simulink model "AirRefueling_Platform_IBVS"  (R2022b)
settings: Solver=FixedStepAuto  StartTime=0.0  StopTime=70  FixedStep=0.02  RelTol=1e-5  AbsTol=1e-4  EnableMultiTasking=on
InitFcn:
  | F16_Init
values from neighbouring files (symbols this model uses):
  airSpeed = 393.720000000000    (= 393.72)    [F16_Init.m]    (also in Initialization.m)
  alpha0 = trimAlpha*180/pi    (= 6.62393794015)    [F16_Init.m]    (also in Initialization.m)
  altitude = 9843    [F16_Init.m]    (also in Initialization.m)
  b_ref = 30.0    (= 30)    [F16_Init.m]    (also in Initialization.m)
  C2m = [C(1,:) ... (first row only)    [F16_Init.m]    (also in Initialization.m)
  d_f_rc = [3.75;0;-0.86]    [F16_Init.m]
  d_pr_rc = [6.06;0.54;-0.86]    [F16_Init.m]
  dLEF = 0    [F16_Init.m]    (also in Initialization.m)
  fi_flag = 1    [F16_Init.m]    (also in Initialization.m)
  Kc = [ ... (first row only)    [F16_Init.m]    (also in Initialization.m)
  Ki = zeros(4,3)    [F16_Init.m]    (also in Initialization.m)
  Kp = zeros(4,18)    [F16_Init.m]    (also in Initialization.m)
  mass = 636.94    [F16_Init.m]    (also in Initialization.m)
  p0_rc = [-14.35-6.06-6;-0.54-(2);5.12+0.86-(-2)]    [F16_Init.m]
  q = zeros(N,1)    [hose3D_n_air_Fv_correction.m]
  trim_ail = 0.00874607850103852    (= 0.00874607850104)    [F16_Init.m]    (also in Initialization.m)
  trim_control = [trim_thrust;trim_ele;trim_ail;trim_rud]    [F16_Init.m]    (also in Initialization.m)
  trim_ele = -2.97973164860638    (= -2.97973164861)    [F16_Init.m]    (also in Initialization.m)
  trim_rud = 0.0680302158182712    (= 0.0680302158183)    [F16_Init.m]    (also in Initialization.m)
  trim_state1 = [trim_state;0;0;0;0;0;0]    [F16_Init.m]    (also in Initialization.m)
  trim_thrust = 2279.08519954656    (= 2279.08519955)    [F16_Init.m]    (also in Initialization.m)
undefined symbols (not defined in the file or in its folder): F, gray, MIL, vt0
libraries: aerolibconvert2 x4, aerolibasang x4, aerolibwind2 x3, visionmorphops x3, vrlib x2, aerolibobsolete x2, simulink x1, visionconversions x1, visiongeotforms x1, aerolibatmos2 x1, aerolibadyn x1, aerolibanimutils x1
(part 1 of 2)
settings Model: Creator=WhisPer  LastModifiedBy=Jinrui
settings SolverCC: AutoScaleAbsTol=off  AlgebraicLoopSolver=TrustRegion
settings DataIOCC: LimitDataPoints=on  SaveFormat=Array  ReturnWorkspaceOutputs=off
settings OptimizationCC: LifeSpan=inf
settings DebuggingCC: UnderspecifiedInitializationDetection=Classic  MergeDetectMultiDrivingBlocksExec=none  SolverPrmCheckMsg=warning  UnconnectedInputMsg=warning  UnconnectedOutputMsg=warning  UnconnectedLineMsg=warning  StateNameClashWarn=warning  SFUnexpectedBacktrackingDiag=warning  SFNoUnconditionalDefaultTransitionDiag=warning  SFExecutionAtInitializationDiag=none  SFMachineParentedDataDiag=warning  ArithmeticOperatorsInVariantConditions=warning
settings HardwareCC: ProdBitPerPointer=32  ProdBitPerSizeT=32  ProdBitPerPtrDiffT=32  ProdLargestAtomicFloat=None  ProdIntDivRoundTo=Undefined  ProdEndianess=Unspecified  ProdWordSize=32  ProdHWDeviceType=32-bit Generic
settings ModelReferenceCC: EnableRefExpFcnMdlSchedulingChecks=on  PropagateSignalLabelsOutOfModel=off
settings SFSimCC: SimUseLocalCustomCode=off  CustomCodeUndefinedFunction=UseInterfaceOnly
settings RTWCC: RTWUseLocalCustomCode=off  DLArmComputeVersion=19.05
settings CodeAppCC: StateflowObjectComments=on
settings GRTTargetCC: TargetLangStandard=C89/C90 (ANSI)
settings ConfigComp: CovMetricSettings=dw  CovSaveCumulativeToWorkspaceVar=on  CovSaveSingleToWorkspaceVar=on  CovExternalEMLEnable=off

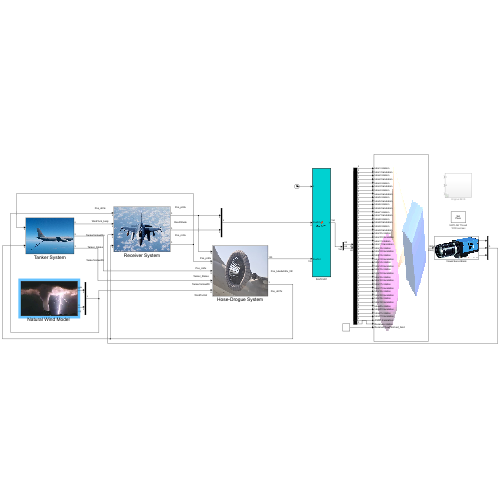
[thumbnail: Simulink's stored preview of the top-level diagram]
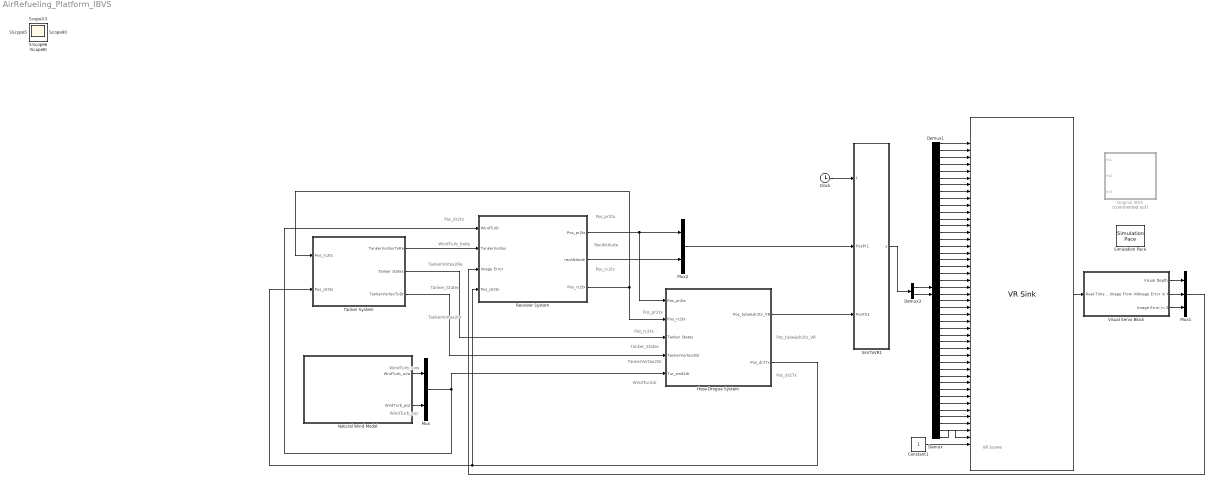
== system AirRefueling_Platform_IBVS ==
  note: Pos_pr2tx
  note: VR Scene
  note: RecAttitude
  note: WindTurb_uvw
  note: WindTurb_pqr
  note: Pos_dr2Tx
  note: Pos_tube&dr2tx_VR
  note: WindTur2dr
  note: Pos_pr2tx
  note: WindTurb_body
  note: Pos_dr2tx
  note: Pos_rc2tx
  note: TankerVortex2Re
  note: TankerVortex2Dr
  note: Tanker_States
  note: Tanker_States
  note: TankerVortex2Dr
  note: Pos_rc2tx
  " " : vrlib/VR Sink  InstantiateOnLoad=on  SampleTime=-1  ViewEnable=on  RemoteChange=off  RemoteView=off  FieldsWritten=tube1.rotation.4.1.1.double#tube1.translation.3.1.1.double#tube2.rotation.4.1.1.double#tube2.translation.3.1.1.double#tube3.rotation.4.1.1.double#tube3.translation.3.1.1.double#tube4.rotation.4.1.1.double#tube4.translation.3.1.1.double#tube5.rotation.4.1.1.double#tube5.translation.3.1.1.double#tube6.rotation.4.1.1.double#tube6.translation.3.1.1.double#tube7.rotation.4.1.1.double#tube7.translation.3.1.1.double#tube8.rotation.4.1.1.double#tube8.translation.3.1.1.double#tube9.rotation.4.1.1.double#tube9.translation.3.1.1.double#tube10.rotation.4.1.1.double#tube10.translation.3.1.1.double#tube11.rotation.4.1.1.double#tube11.translation.3.1.1.double#tube12.rotation.4.1.1.double#tube12.translation.3.1.1.double#tube13.rotation.4.1.1.double#tube13.translation.3.1.1.double#tube14.rotation.4.1.1.double#tube14.translation.3.1.1.double#tube15.rotation.4.1.1.double#tube15.translation.3.1.1.double#tube16.rotation.4.1.1.double#tube16.translation.3.1.1.double#tube17.rotation.4.1.1.double#tube17.translation.3.1.1.double#tube18.rotation.4.1.1.double#tube18.translation.3.1.1.double#tube19.rotation.4.1.1.double#tube19.translation.3.1.1.double#tube20.rotation.4.1.1.double#tube20.translation.3.1.1.double#tube21.rotation.4.1.1.double#tube21.translation.3.1.1.double#ASDD.translation.3.1.1.double#Receiver.rotation.4.1.1.double#ReceiverViewPoint.set_bind.1.1.1.logical  WorldFileName=AirRefuelingTubeSim_Image.WRL  AutoView=off  VideoDimensions=[200 320]  AllowVariableSize=off  FigureProperties="{'Position', 'Name', 'Viewpoint', 'CameraBound', 'CameraDirection', 'CameraPosition', 'CameraUpVector', 'ZoomFactor', 'Antialiasing', 'Headlight', 'Lighting', 'NavPanel', 'Sound', 'StatusBar', 'Stereo3D', 'Stereo3DCameraOffset', 'Stereo3DHIT', 'ToolBar', 'Textures', 'Transparency', 'Triad', 'Wireframe', 'NavZones', 'NavMode', 'NavSpeed', 'CaptureFileFormat', 'CaptureFileName', 'Record2DCompressMethod', 'Record2DCompressQuality', 'Record2D', 'Record2DFileName', 'Record2DFPS'; [3.0000000000000000e+01   6.0000000000000000e+01   3.2000000000000000e+02   2.0000000000000000e+02], '', 'Receive1', 'on', [-9.4108294567116141e-02   0.0000000000000000e+00  -9.9556196637560879e-01], [-2.1616954617207307e-01   0.0000000000000000e+00  -1.0387194196845528e+00], [0.0000000000000000e+00   1.0000000000000000e+00   0.0000000000000000e+00], [1.0000000000000000e+00], 'on', 'on', 'on', 'none', 'on', 'off', 'off', [1.0000000149011612e-01], [0.0000000000000000e+00], 'off', 'on', 'on', 'none', 'off', 'off', 'walk', 'normal', 'tif', '%f_anim_%n.tif', 'auto', [7.5000000000000000e+01], 'off', '***video***', 'auto'}"
  Clock : Clock
  Constant1 : Constant
  Demux : Demux  Outputs=22
  Demux1 : Demux  Outputs=22
  Demux3 : Demux  Outputs=[88,66]
  Hose-Drogue System : Subsystem
      mask Display: image(imread('Icon\drogue.jpg'))
  Mux : Mux  Inputs=2
  Mux1 : Mux  Inputs=3
  Mux2 : Mux  Inputs=2
  "Natural Wind Model " : Subsystem
      mask Display: image(imread('Icon\Enviroment.jpg'))
  Original IBVS : Subsystem  Commented=on
  Receiver System : Subsystem
      mask Display: image(imread('Icon\f16thumb.jpg'))
  SimToVR1 : MATLAB Function  TreatAsAtomicUnit=on
  Simulation Pace : aerolibanimutils/Simulation Pace  SimulationPace=1000  SleepMode=MATLAB Thread  OutputPaceError=off  SampleTime=-1
  Tanker System : Subsystem
      mask Display: image(imread('Icon\tanker.jpg'))
  Visual Servo Block : Subsystem
      mask Display: image('icon/camera.jpg');
  Scope{,1,3..34} (34 alike) : Scope
  wires:
  Receiver System/1(Pos_pr2tx) -> Mux2/1, Hose-Drogue System/1(Pos_pr2tx)
  Hose-Drogue System/2(Pos_dr2Tx) -> Tanker System/2(Pos_dr2tx), Receiver System/4(Pos_dr2tx)
  Mux/1 -> Receiver System/1(WindTurb), Hose-Drogue System/5(Tur_wnd2dr)
  Receiver System/2(recAttitude) -> Mux2/2
  Hose-Drogue System/1(Pos_tube&dr2tx_VR) -> SimToVR1/3(PosTb1)
  Mux2/1 -> SimToVR1/2(PosPr1)
  "Natural Wind Model "/1(WndTurb_uvw) -> Mux/1
  "Natural Wind Model "/2(WndTurb_pqr) -> Mux/2
  Demux3/2 -> Demux/1
  Demux/22 -> " "/43
  Demux1/22 -> " "/44
  Demux3/1 -> Demux1/1
  Tanker System/2(Tanker states) -> Hose-Drogue System/3(Tanker States)
  Tanker System/3(TankerVortexToDr) -> Hose-Drogue System/4(TankerVortex2Dr)
  Tanker System/1(TankerVortexToRe) -> Receiver System/2(TankerVortex)
  Receiver System/3(Pos_rc2tx) -> Tanker System/1(Pos_rc2tx), Hose-Drogue System/2(Pos_rc2tx)
  Clock/1 -> SimToVR1/1(t)
  Demux1/1 -> " "/1
  Demux/1 -> " "/2
  Demux1/2 -> " "/3
  Demux/2 -> " "/4
  Demux1/3 -> " "/5
  Demux/3 -> " "/6
  Demux1/4 -> " "/7
  Demux/4 -> " "/8
  Demux1/5 -> " "/9
  Demux/5 -> " "/10
  Demux1/6 -> " "/11
  Demux/6 -> " "/12
  Demux1/7 -> " "/13
  Demux/7 -> " "/14
  Demux1/8 -> " "/15
  Demux/8 -> " "/16
  Demux1/9 -> " "/17
  Demux/9 -> " "/18
  Demux1/10 -> " "/19
  Demux/10 -> " "/20
  Demux1/11 -> " "/21
  Demux/11 -> " "/22
  Demux1/12 -> " "/23
  Demux/12 -> " "/24
  Demux1/13 -> " "/25
  Demux/13 -> " "/26
  Demux1/14 -> " "/27
  Demux/14 -> " "/28
  Demux1/15 -> " "/29
  Demux/15 -> " "/30
  Demux1/16 -> " "/31
  Demux/16 -> " "/32
  Demux1/17 -> " "/33
  Demux/17 -> " "/34
  Demux1/18 -> " "/35
  Demux/18 -> " "/36
  Demux1/19 -> " "/37
  Demux/19 -> " "/38
  Demux1/20 -> " "/39
  Demux/20 -> " "/40
  Demux1/21 -> " "/41
  Demux/21 -> " "/42
  Constant1/1 -> " "/45
  " "/1 -> Visual Servo Block/1(Real-Time Image From VR)
  Visual Servo Block/1(Visual Depth) -> Mux1/1
  Visual Servo Block/2(Image Error in Y) -> Mux1/2
  Visual Servo Block/3(Image Error in Z) -> Mux1/3
  Mux1/1 -> Receiver System/3(Image Error)
  SimToVR1/1(y) -> Demux3/1

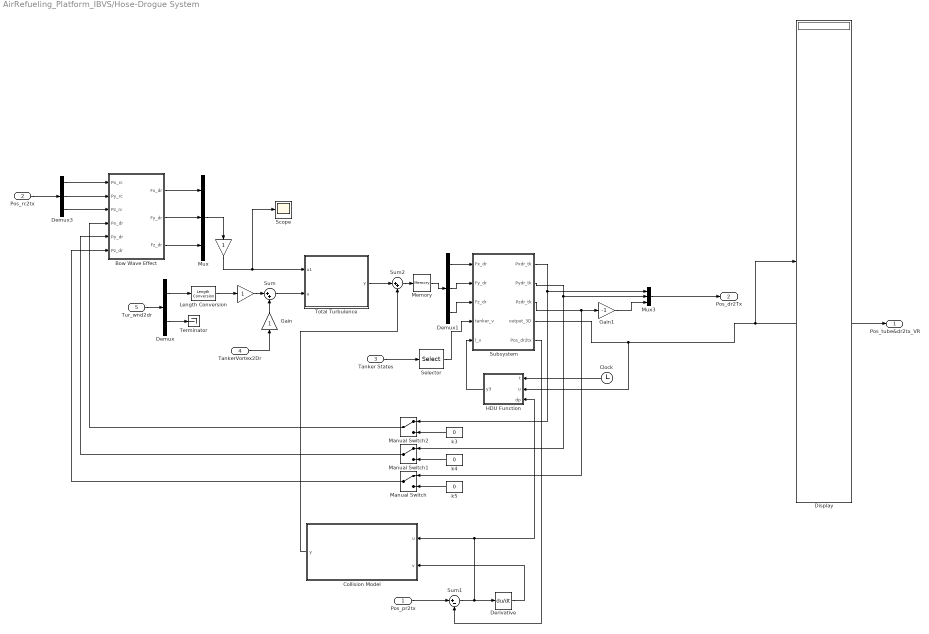
== system AirRefueling_Platform_IBVS/Hose-Drogue System ==
  Pos_pr2tx : Inport
  Pos_rc2tx : Inport  Port=2
  Tanker States : Inport  Port=3
  TankerVortex2Dr : Inport  Port=4
  Tur_wnd2dr : Inport  Port=5
  " " : Gain
  "  " : Gain
  Bow Wave Effect : Subsystem
  Clock : Clock
  Collision Model : MATLAB Function  TreatAsAtomicUnit=on
  Demux : Demux  Outputs=2
  Demux1 : Demux  Outputs=3
  Demux3 : Demux  Outputs=3
  Derivative : Derivative
  Display : Display
  Gain : Gain
  Gain1 : Gain  Gain=-1
  HDU Function : MATLAB Function  TreatAsAtomicUnit=on
  Length Conversion : aerolibconvert2/Length Conversion  IU=ft  OU=m
  Manual Switch : ManualSwitch
  Manual Switch1 : ManualSwitch
  Manual Switch2 : ManualSwitch
  Memory : Memory
  Mux : Mux  Inputs=3
  Mux3 : Mux  Inputs=3
  Scope : Scope
  Selector : Selector  InputPortWidth=9  IndexOptions=Index vector (dialog)  Indices=[4 5 6]  OutputSizes=1
  Subsystem : Subsystem
  Sum : Sum  Inputs=|++
  Sum1 : Sum  Inputs=|+-
  Sum2 : Sum  Inputs=|++
  Terminator : Terminator
  "Total Turbulence  " : MATLAB Function  TreatAsAtomicUnit=on
  k3 : Constant  Value=0
  k4 : Constant  Value=0
  k5 : Constant  Value=0
  Pos_tube&dr2tx_VR : Outport
  Pos_dr2Tx : Outport  Port=2
  wires:
  Mux/1 -> "  "/1
  TankerVortex2Dr/1 -> Gain/1
  Demux/1 -> Length Conversion/1
  Demux1/3 -> Subsystem/3(Fz_dr)
  Demux1/2 -> Subsystem/2(Fy_dr)
  Demux1/1 -> Subsystem/1(Fx_dr)
  Demux/2 -> Terminator/1
  Tur_wnd2dr/1 -> Demux/1
  Pos_rc2tx/1 -> Demux3/1
  Bow Wave Effect/3(Fz_dr) -> Mux/3
  Sum/1 -> "Total Turbulence  "/2(u)
  Bow Wave Effect/2(Fy_dr) -> Mux/2
  Bow Wave Effect/1(Fx_dr) -> Mux/1
  Demux3/1 -> Bow Wave Effect/1(Px_rc)
  k4/1 -> Manual Switch1/2
  Manual Switch1/1 -> Bow Wave Effect/5(Py_dr)
  Manual Switch2/1 -> Bow Wave Effect/4(Px_dr)
  k5/1 -> Manual Switch/2
  k3/1 -> Manual Switch2/2
  Mux3/1 -> Pos_dr2Tx/1
  Manual Switch/1 -> Bow Wave Effect/6(Pz_dr)
  Subsystem/2(Pydr_tk) -> Manual Switch1/1, Mux3/2
  Subsystem/1(Pxdr_tk) -> Manual Switch2/1, Mux3/1
  Gain1/1 -> Mux3/3
  Subsystem/3(Pzdr_tk) -> Gain1/1, Manual Switch/1
  Demux3/3 -> Bow Wave Effect/3(Pz_rc)
  Demux3/2 -> Bow Wave Effect/2(Py_rc)
  "Total Turbulence  "/1(y) -> Sum2/1
  Subsystem/4(output_3D) -> Display/1, Pos_tube&dr2tx_VR/1, HDU Function/2(u)
  Gain/1 -> Sum/2
  " "/1 -> Sum/1
  "  "/1 -> Scope/1, "Total Turbulence  "/1(u1)
  Length Conversion/1 -> " "/1
  Tanker States/1 -> Selector/1
  Sum1/1 -> HDU Function/3(dp), Collision Model/1(u), Derivative/1
  Derivative/1 -> Collision Model/2(v)
  Sum2/1 -> Memory/1
  Collision Model/1(y) -> Sum2/2
  Selector/1 -> Subsystem/4(tanker_v)
  Subsystem/5(Pos_dr2tx) -> Sum1/2
  Memory/1 -> Demux1/1
  Clock/1 -> HDU Function/1(t)
  HDU Function/1(y3) -> Subsystem/5(l_v)
  Pos_pr2tx/1 -> Sum1/1

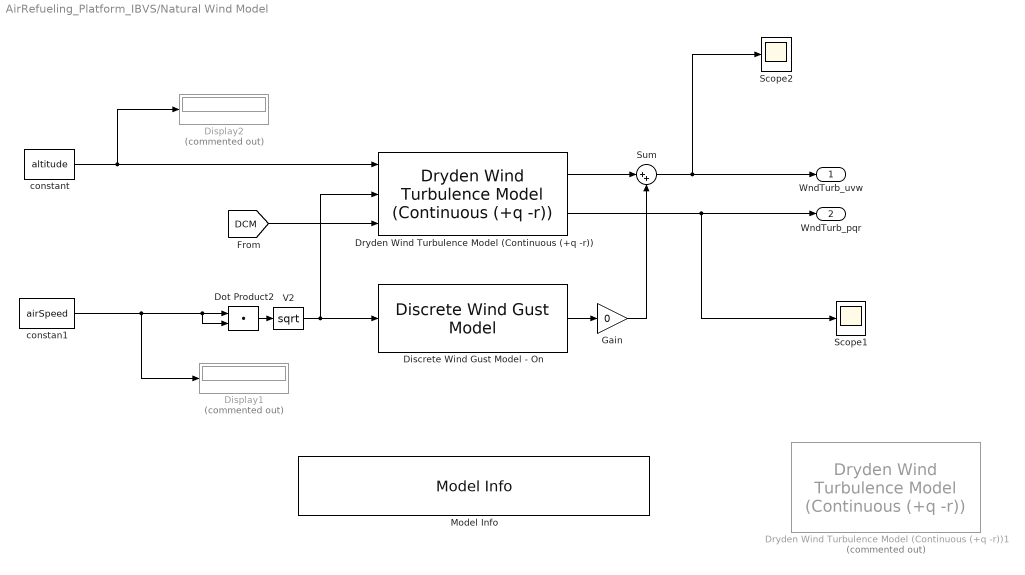
== system AirRefueling_Platform_IBVS/Natural Wind Model  ==
  Discrete Wind Gust Model - On : aerolibwind2/Discrete Wind Gust Model  units=English (Velocity in ft/s)  Gx=on  Gy=on  Gz=on  t_0=20  d_m=[120 120 80]  v_m=[0 0 0]
  Display1 : Display  Commented=on
  Display2 : Display  Commented=on
  Dot Product2 : DotProduct  SaturateOnIntegerOverflow=on  InputSameDT=off  OutDataTypeStr=Inherit: Inherit via internal rule
  Dryden Wind Turbulence Model (Continuous (+q -r)) : aerolibwind2/Dryden Wind Turbulence Model  (Continuous (+q -r))  units=English (Velocity in ft/s)  spec=MIL-F-8785C  model=Continuous Dryden (+q -r)  W20=5  Wdeg=0  TurbProb=2x10^-1  L_high=533.4  Wingspan=4  ts=0.02  Seed=[23341 23342 23343 23344]  T_on=on
  Dryden Wind Turbulence Model (Continuous (+q -r))1 : aerolibwind2/Dryden Wind Turbulence Model  (Continuous (+q -r))  Commented=on  units=English (Velocity in ft/s)  spec=MIL-F-8785C  model=Continuous Dryden (+q -r)  W20=5  Wdeg=0  TurbProb=2x10^-1  L_high=533.5  Wingspan=6  ts=0.02  Seed=1+fix(3650*rand(1,4))  T_on=on
  Gain : Gain  Gain=0
  Model Info : simulink/Model-Wide Utilities/Model Info  Frame=on  DisplayStringWithTags=|  HorizontalTextAlignment=Center  LeftAlignmentValue=0.5
      | The resultant mean wind speed and angular rates is in the body-fixed axis. 
      | The simulation parameter is set to
      | altitude:3000m
      | airspeed:120m/s
  Scope1 : Scope
  Scope2 : Scope
  Sum : Sum  Inputs=|++  InputSameDT=on  SaturateOnIntegerOverflow=on  OutDataTypeStr=Inherit: Same as first input
  V2 : Math  Operator=sqrt  SignedPower=on
  constan1 : Constant  Value=airSpeed
  constant : Constant  Value=altitude
  WndTurb_uvw : Outport
  WndTurb_pqr : Outport  Port=2
  wires:
  V2/1 -> Dryden Wind Turbulence Model (Continuous (+q -r))/2, Discrete Wind Gust Model - On/1
  Dot Product2/1 -> V2/1
  constan1/1 -> Dot Product2/1, Dot Product2/2, Display1/1
  Discrete Wind Gust Model - On/1 -> Gain/1
  Dryden Wind Turbulence Model (Continuous (+q -r))/1 -> Sum/1
  constant/1 -> Dryden Wind Turbulence Model (Continuous (+q -r))/1, Display2/1
  [DCM] -> Dryden Wind Turbulence Model (Continuous (+q -r))/3
  Sum/1 -> WndTurb_uvw/1, Scope2/1
  Dryden Wind Turbulence Model (Continuous (+q -r))/2 -> Scope1/1, WndTurb_pqr/1
  Gain/1 -> Sum/2

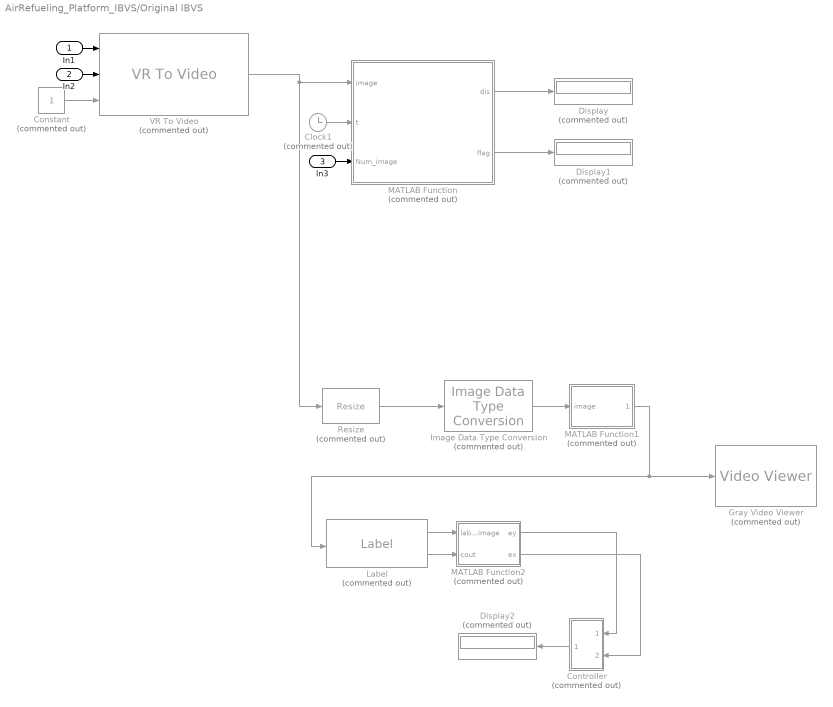
== system AirRefueling_Platform_IBVS/Original IBVS ==
  In1 : Inport
  In2 : Inport  Port=2
  In3 : Inport  Port=3
  Clock1 : Clock  Commented=on
  Constant : Constant  Commented=on
  Controller : Subsystem  Commented=on
  Display : Display  Commented=on
  Display1 : Display  Commented=on
  Display2 : Display  Commented=on
  Gray Video Viewer : VideoViewer  Commented=on  FigPos=[594 894 615 423]
  Image Data Type Conversion : visionconversions/Image Data Type Conversion  Commented=on  outDT=double  isSigned=on  wordLen=16  numFracBits=0
  Label : visionmorphops/Label  Commented=on  conn=8  output=Label matrix and number of labels  outType=Automatic  lastLabel=maximum value of the output data type
  MATLAB Function : MATLAB Function  Commented=on  TreatAsAtomicUnit=on
  MATLAB Function1 : MATLAB Function  Commented=on  TreatAsAtomicUnit=on
  MATLAB Function2 : MATLAB Function  Commented=on  TreatAsAtomicUnit=on
  Resize : visiongeotforms/Resize  Commented=on  specify=Output size as a percentage of input size  rfactor=[200 150]  outCols=25  outRows=25  outRowsCols=[25 35]  interp_method=Bilinear  antialias=on  useROI=off  roiFlag=off  prodOutputMode=Binary point scaling  prodOutputWordLength=32  prodOutputFracLength=10  roundingMode=Nearest  overflowMode=on
  VR To Video : vrlib/VR To Video  Commented=on  InstantiateOnLoad=on  SampleTime=0.01  ViewEnable=on  RemoteChange=off  RemoteView=off  FieldsWritten=Anigroup-1-Intrp7-transform.rotation.4.1.1.double#Anigroup-1-Intrp7-transform.translation.3.1.1.double#ReceiverViewPoint.set_bind.1.1.1.logical  WorldFileName=AirRefuelingTubeSim.WRL  AutoView=off  VideoDimensions=[200 320]  AllowVariableSize=off  FigureProperties="{'Position', 'Name', 'Viewpoint', 'CameraBound', 'CameraDirection', 'CameraPosition', 'CameraUpVector', 'ZoomFactor', 'Antialiasing', 'Headlight', 'Lighting', 'NavPanel', 'Sound', 'StatusBar', 'Stereo3D', 'Stereo3DCameraOffset', 'Stereo3DHIT', 'ToolBar', 'Textures', 'Transparency', 'Triad', 'Wireframe', 'NavZones', 'NavMode', 'NavSpeed', 'CaptureFileFormat', 'CaptureFileName', 'Record2DCompressMethod', 'Record2DCompressQuality', 'Record2D', 'Record2DFileName', 'Record2DFPS'; [3.0000000000000000e+01   6.0000000000000000e+01   3.2000000000000000e+02   2.0000000000000000e+02], '', 'Receive1', 'on', [0.0000000000000000e+00   0.0000000000000000e+00  -1.0000000000000000e+00], [0.0000000000000000e+00   0.0000000000000000e+00   0.0000000000000000e+00], [0.0000000000000000e+00   1.0000000000000000e+00   0.0000000000000000e+00], [1.0000000000000000e+00], 'on', 'on', 'on', 'none', 'on', 'off', 'off', [1.0000000149011612e-01], [0.0000000000000000e+00], 'off', 'on', 'on', 'none', 'off', 'off', 'walk', 'normal', 'tif', '%f_anim_%n.tif', 'auto', [7.5000000000000000e+01], 'off', '***video***', 'auto'}"
  wires:
  MATLAB Function/2(flag) -> Display1/1
  MATLAB Function/1(dis) -> Display/1
  VR To Video/1 -> MATLAB Function/1(image), Resize/1
  Clock1/1 -> MATLAB Function/2(t)
  Resize/1 -> Image Data Type Conversion/1
  Image Data Type Conversion/1 -> MATLAB Function1/1(image)
  MATLAB Function1/1(bw_image) -> Label/1, Gray Video Viewer/1
  Label/1 -> MATLAB Function2/1(label_image)
  Label/2 -> MATLAB Function2/2(cout)
  MATLAB Function2/1(ey) -> Controller/1(In1)
  MATLAB Function2/2(ex) -> Controller/2(In2)
  Controller/1(Out2) -> Display2/1
  Constant/1 -> VR To Video/3
  In2/1 -> VR To Video/2
  In1/1 -> VR To Video/1
  In3/1 -> MATLAB Function/3(Num_image)

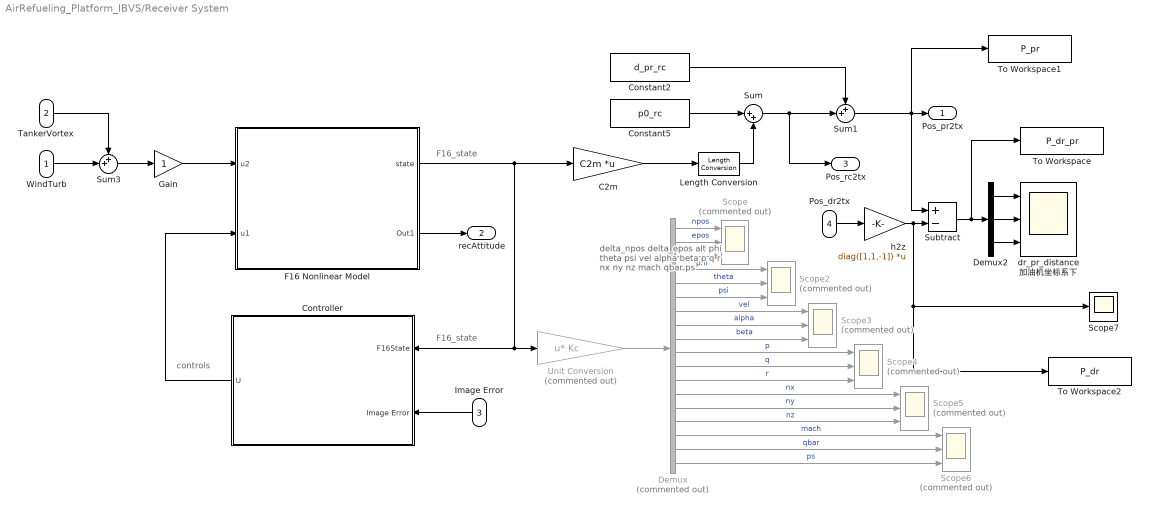
== system AirRefueling_Platform_IBVS/Receiver System ==
  note: controls
  note: F16_state
  note: delta_npos
      | delta_epos
      | alt
      | phi
      | theta
      | psi
      | vel
      | alpha
      | beta
      | p
      | q
      | r
      | nx
      | ny
      | nz
      | mach
      | qbar
      | ps
  note: F16_state
  WindTurb : Inport
  TankerVortex : Inport  Port=2
  Image Error : Inport  Port=3
  Pos_dr2tx : Inport  Port=4
  C2m : Gain  Gain=C2m  Multiplication=Matrix(K*u) (u vector)
  Constant2 : Constant  Value=d_pr_rc
  Constant5 : Constant  Value=p0_rc
  Controller : Subsystem
      mask Display: image(imread('Icon\F16_Pilot.jpg'))
  Demux : Demux  Commented=on  Outputs=18
      settings: DisplayOption=none
  Demux2 : Demux  Outputs=3
  F16 Nonlinear Model : Subsystem
      mask Display: image(imread('Icon\fighter_f16.jpg'))
  Gain : Gain
  Length Conversion : aerolibconvert2/Length Conversion  IU=ft  OU=m
  Scope{,2..6} (6 alike) : Scope  Commented=on  NumInputPorts=3
  Scope7 : Scope
  Subtract : Sum  Inputs=+-
  Sum : Sum  Inputs=|++
  Sum1 : Sum  Inputs=++|
  Sum3 : Sum  Inputs=++|
  To Workspace : ToWorkspace  VariableName=P_dr_pr  SampleTime=-1
  To Workspace1 : ToWorkspace  VariableName=P_pr  SampleTime=-1
  To Workspace2 : ToWorkspace  VariableName=P_dr  SampleTime=-1
  Unit Conversion : Gain  Commented=on  Gain=Kc  Multiplication=Matrix(u*K)
  dr_pr_distance 加油机坐标系下 : Scope  NumInputPorts=3
  h2z : Gain  Gain=diag([1,1,-1])  Multiplication=Matrix(K*u)
  Pos_pr2tx : Outport
  recAttitude : Outport  Port=2
  Pos_rc2tx : Outport  Port=3
  wires:
  Controller/1(U) -> F16 Nonlinear Model/2(u1)
  WindTurb/1 -> Sum3/2
  Demux/1 -> Scope/1  "npos"
  Demux/2 -> Scope/2  "epos"
  Demux/3 -> Scope/3  "alt"
  Demux/5 -> Scope2/2  "theta"
  Demux/6 -> Scope2/3  "psi"
  Demux/7 -> Scope3/1  "vel"
  Demux/8 -> Scope3/2  "alpha"
  Demux/9 -> Scope3/3  "beta"
  Demux/10 -> Scope4/1  "p"
  Demux/11 -> Scope4/2  "q"
  Demux/12 -> Scope4/3  "r"
  Demux/13 -> Scope5/1  "nx"
  Demux/14 -> Scope5/2  "ny"
  Demux/15 -> Scope5/3  "nz"
  Demux/4 -> Scope2/1  "phi"
  Demux/16 -> Scope6/1  "mach"
  Demux/17 -> Scope6/2  "qbar"
  Demux/18 -> Scope6/3  "ps"
  Unit Conversion/1 -> Demux/1
  F16 Nonlinear Model/2(Out1) -> recAttitude/1
  C2m/1 -> Length Conversion/1
  Sum3/1 -> Gain/1
  TankerVortex/1 -> Sum3/1
  Length Conversion/1 -> Sum/2
  Constant5/1 -> Sum/1
  Sum1/1 -> Subtract/1, To Workspace1/1, Pos_pr2tx/1
  Sum/1 -> Pos_rc2tx/1, Sum1/2
  Constant2/1 -> Sum1/1
  Image Error/1 -> Controller/2(Image Error)
  Gain/1 -> F16 Nonlinear Model/1(u2)
  h2z/1 -> To Workspace2/1, Scope7/1, Subtract/2
  Pos_dr2tx/1 -> h2z/1
  Subtract/1 -> To Workspace/1, Demux2/1
  F16 Nonlinear Model/1(state) -> C2m/1, Controller/1(F16State), Unit Conversion/1
  Demux2/2 -> dr_pr_distance 加油机坐标系下/2
  Demux2/1 -> dr_pr_distance 加油机坐标系下/1
  Demux2/3 -> dr_pr_distance 加油机坐标系下/3

== system AirRefueling_Platform_IBVS/Tanker System ==
  note: pt
  note: vt
  note: al
  Pos_rc2tx : Inport
  Pos_dr2tx : Inport  Port=2
  " " : MATLAB Function  TreatAsAtomicUnit=on
  "  " : MATLAB Function  TreatAsAtomicUnit=on
  Demux : Demux  Outputs=2
  Integrator : Integrator  InitialCondition=vt0
  Integrator1 : Integrator  InitialCondition=[0;0;0]
  Length Conversion : aerolibconvert2/Length Conversion  IU=m  OU=ft
  Mux : Mux  Inputs=3
  Mux1 : Mux  Inputs=2
  tanker acceleration : Constant  Value=[0;0;0]
  TankerVortexToRe : Outport
  Tanker states : Outport  Port=2
  TankerVortexToDr : Outport  Port=3
  wires:
  tanker acceleration/1 -> Mux/3, Integrator/1
  Integrator/1 -> Mux/2, Integrator1/1
  Mux/1 -> Tanker states/1
  Pos_rc2tx/1 -> " "/1(u)
  Pos_dr2tx/1 -> "  "/1(u)
  "  "/1(y) -> TankerVortexToDr/1
  Integrator1/1 -> Mux/1
  " "/1(y) -> Demux/1
  Mux1/1 -> TankerVortexToRe/1
  Demux/2 -> Mux1/2
  Length Conversion/1 -> Mux1/1
  Demux/1 -> Length Conversion/1

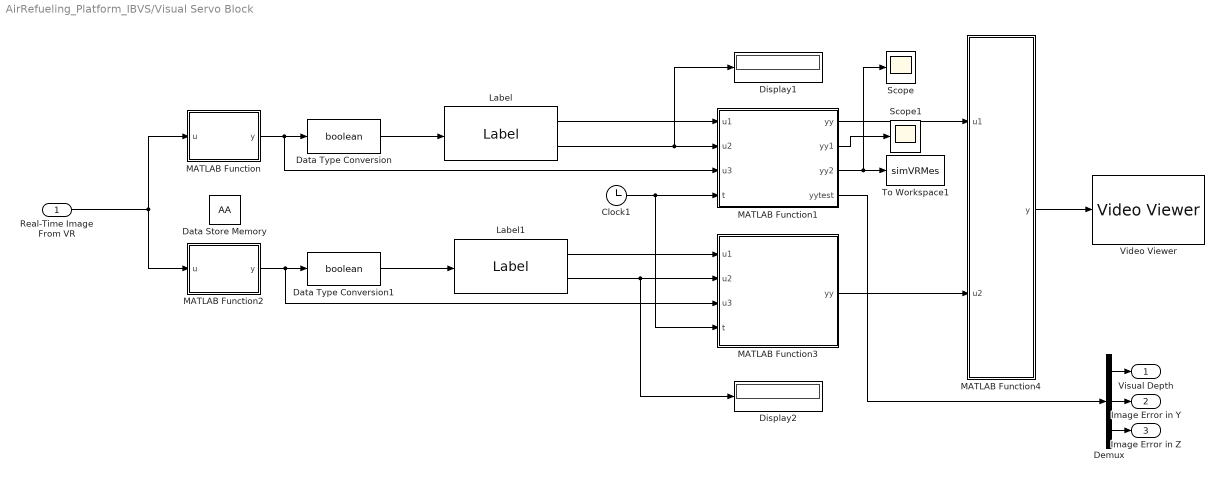
== system AirRefueling_Platform_IBVS/Visual Servo Block ==
  Real-Time Image From VR : Inport
  Clock1 : Clock
  Data Store Memory : DataStoreMemory  DataStoreName=AA  InitialValue=[0 0 0]  ShowAdditionalParam=off  OutDataTypeStr=double
  Data Type Conversion : DataTypeConversion  OutDataTypeStr=boolean  SaturateOnIntegerOverflow=off  RndMeth=Floor
  Data Type Conversion1 : DataTypeConversion  OutDataTypeStr=boolean  SaturateOnIntegerOverflow=off  RndMeth=Floor
  Demux : Demux  Outputs=3
  Display1 : Display
  Display2 : Display
  Label : visionmorphops/Label  conn=8  output=Label matrix and number of labels  outType=Automatic  lastLabel=maximum value of the output data type
  Label1 : visionmorphops/Label  conn=8  output=Label matrix and number of labels  outType=Automatic  lastLabel=maximum value of the output data type
  MATLAB Function : MATLAB Function  TreatAsAtomicUnit=on
  MATLAB Function1 : MATLAB Function  TreatAsAtomicUnit=on
  MATLAB Function2 : MATLAB Function  TreatAsAtomicUnit=on
  MATLAB Function3 : MATLAB Function  TreatAsAtomicUnit=on
  MATLAB Function4 : MATLAB Function  TreatAsAtomicUnit=on
  Scope : Scope
  Scope1 : Scope
  To Workspace1 : ToWorkspace  VariableName=simVRMes  SampleTime=-1
  Video Viewer : VideoViewer  colormapValue=gray(256)  FigPos=[481 840 1101 615]
  Visual Depth : Outport
  Image Error in Y : Outport  Port=2
  Image Error in Z : Outport  Port=3
  wires:
  Real-Time Image From VR/1 -> MATLAB Function/1(u), MATLAB Function2/1(u)
  Label/1 -> MATLAB Function1/1(u1)
  MATLAB Function/1(y) -> MATLAB Function1/3(u3), Data Type Conversion/1
  Data Type Conversion/1 -> Label/1
  MATLAB Function2/1(y) -> MATLAB Function3/3(u3), Data Type Conversion1/1
  Data Type Conversion1/1 -> Label1/1
  Label1/1 -> MATLAB Function3/1(u1)
  Label1/2 -> Display2/1, MATLAB Function3/2(u2)
  MATLAB Function1/1(yy) -> MATLAB Function4/1(u1)
  MATLAB Function3/1(yy) -> MATLAB Function4/2(u2)
  MATLAB Function4/1(y) -> Video Viewer/1
  Clock1/1 -> MATLAB Function3/4(t), MATLAB Function1/4(t)
  Label/2 -> Display1/1, MATLAB Function1/2(u2)
  MATLAB Function1/4(yytest) -> Demux/1
  Demux/1 -> Visual Depth/1
  Demux/2 -> Image Error in Y/1
  Demux/3 -> Image Error in Z/1
  MATLAB Function1/3(yy2) -> Scope/1, To Workspace1/1
  MATLAB Function1/2(yy1) -> Scope1/1

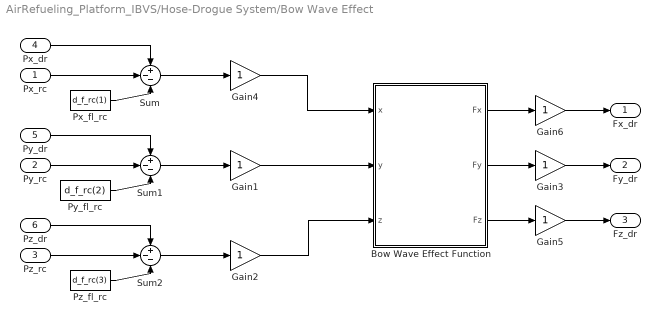
== system AirRefueling_Platform_IBVS/Hose-Drogue System/Bow Wave Effect ==
  Px_rc : Inport
  Py_rc : Inport  Port=2
  Pz_rc : Inport  Port=3
  Px_dr : Inport  Port=4
  Py_dr : Inport  Port=5
  Pz_dr : Inport  Port=6
  Bow Wave Effect Function : MATLAB Function  TreatAsAtomicUnit=on
  Gain{1..6} (6 alike) : Gain
  Px_fl_rc : Constant  Value=d_f_rc(1)
  Py_fl_rc : Constant  Value=d_f_rc(2)
  Pz_fl_rc : Constant  Value=d_f_rc(3)
  Sum : Sum  Inputs=+--
  Sum1 : Sum  Inputs=+--
  Sum2 : Sum  Inputs=+--
  Fx_dr : Outport
  Fy_dr : Outport  Port=2
  Fz_dr : Outport  Port=3
  wires:
  Sum2/1 -> Gain2/1
  Sum1/1 -> Gain1/1
  Bow Wave Effect Function/3(Fz) -> Gain5/1
  Bow Wave Effect Function/2(Fy) -> Gain3/1
  Bow Wave Effect Function/1(Fx) -> Gain6/1
  Gain6/1 -> Fx_dr/1
  Gain5/1 -> Fz_dr/1
  Gain3/1 -> Fy_dr/1
  Gain2/1 -> Bow Wave Effect Function/3(z)
  Gain1/1 -> Bow Wave Effect Function/2(y)
  Gain4/1 -> Bow Wave Effect Function/1(x)
  Pz_dr/1 -> Sum2/1
  Pz_fl_rc/1 -> Sum2/3
  Pz_rc/1 -> Sum2/2
  Py_fl_rc/1 -> Sum1/3
  Py_dr/1 -> Sum1/1
  Py_rc/1 -> Sum1/2
  Px_dr/1 -> Sum/1
  Px_fl_rc/1 -> Sum/3
  Px_rc/1 -> Sum/2
  Sum/1 -> Gain4/1

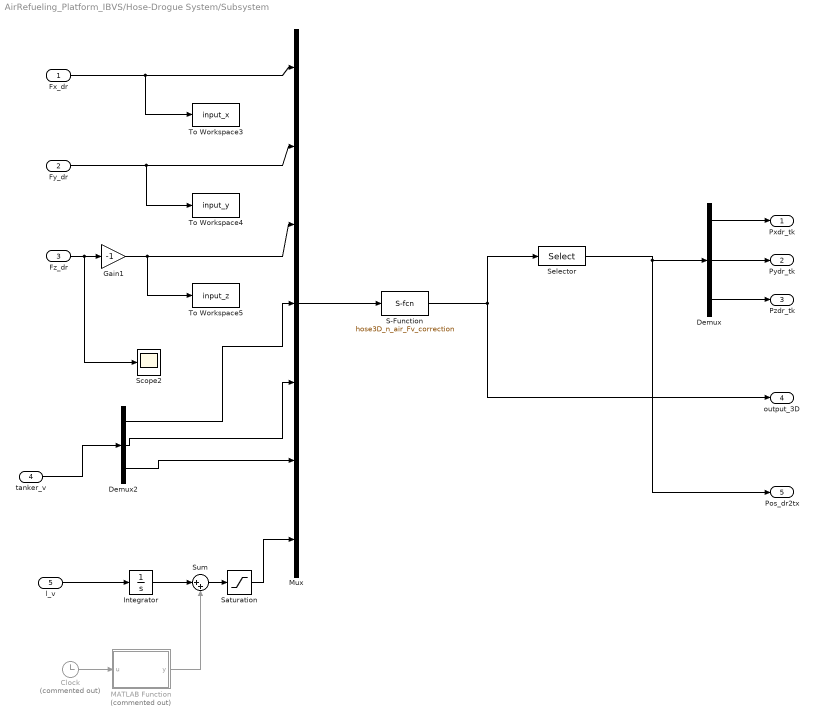
== system AirRefueling_Platform_IBVS/Hose-Drogue System/Subsystem ==
  Fx_dr : Inport
  Fy_dr : Inport  Port=2
  Fz_dr : Inport  Port=3
  tanker_v : Inport  Port=4
  l_v : Inport  Port=5
  Clock : Clock  Commented=on
  Demux : Demux  Outputs=3
  Demux2 : Demux  Outputs=3
  Gain1 : Gain  Gain=-1  ParamDataTypeStr=double  OutDataTypeStr=double
  Integrator : Integrator
  MATLAB Function : MATLAB Function  Commented=on  TreatAsAtomicUnit=on
  Mux : Mux  Inputs=7
  S-Function : S-Function  FunctionName=hose3D_n_air_Fv_correction  SFunctionDeploymentMode=off  EnableBusSupport=off
  Saturation : Saturate  UpperLimit=13  LowerLimit=-1
  Scope2 : Scope
  Selector : Selector  InputPortWidth=100  IndexOptions=Index vector (dialog)  Indices=[58 59 60]  OutputSizes=1
  Sum : Sum  Inputs=|++
  To Workspace3 : ToWorkspace  VariableName=input_x  SampleTime=-1
  To Workspace4 : ToWorkspace  VariableName=input_y  SampleTime=-1
  To Workspace5 : ToWorkspace  VariableName=input_z  SampleTime=-1
  Pxdr_tk : Outport
  Pydr_tk : Outport  Port=2
  Pzdr_tk : Outport  Port=3
  output_3D : Outport  Port=4
  Pos_dr2tx : Outport  Port=5
  wires:
  Mux/1 -> S-Function/1
  Demux2/1 -> Mux/4
  Demux2/2 -> Mux/5
  Demux2/3 -> Mux/6
  Fy_dr/1 -> Mux/2, To Workspace4/1
  Fz_dr/1 -> Scope2/1, Gain1/1
  Fx_dr/1 -> To Workspace3/1, Mux/1
  Demux/1 -> Pxdr_tk/1
  Demux/2 -> Pydr_tk/1
  Demux/3 -> Pzdr_tk/1
  Gain1/1 -> Mux/3, To Workspace5/1
  S-Function/1 -> Selector/1, output_3D/1
  l_v/1 -> Integrator/1
  Sum/1 -> Saturation/1
  Integrator/1 -> Sum/1
  Clock/1 -> MATLAB Function/1(u)
  MATLAB Function/1(y) -> Sum/2
  Saturation/1 -> Mux/7
  tanker_v/1 -> Demux2/1
  Selector/1 -> Pos_dr2tx/1, Demux/1

== system AirRefueling_Platform_IBVS/Original IBVS/Controller ==
  In1 : Inport
  In2 : Inport  Port=2
  Display1 : Display
  Display2 : Display
  "controller " : MATLAB Function  TreatAsAtomicUnit=on
  Out2 : Outport
  wires:
  "controller "/1(y) -> Out2/1
  In1/1 -> Display1/1
  In2/1 -> Display2/1

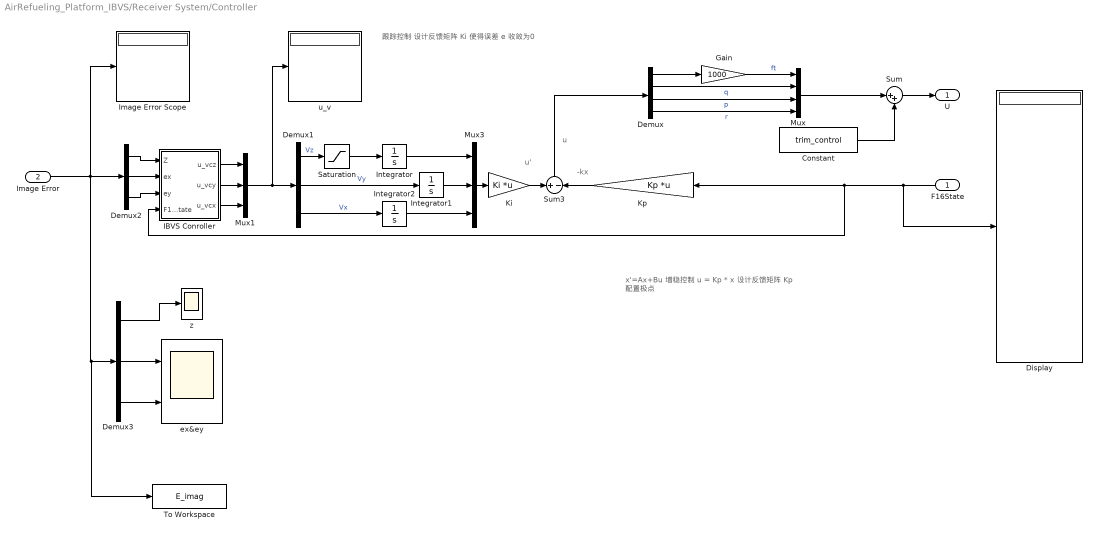
== system AirRefueling_Platform_IBVS/Receiver System/Controller ==
  note: u
  note: -kx
  note: u'
  note: 跟踪控制
      | 设计反馈矩阵 Ki 使得误差 e 收敛为0
  note: x'=Ax+Bu
      | 增稳控制 u = Kp * x
      | 设计反馈矩阵 Kp 配置极点
  F16State : Inport
  Image Error : Inport  Port=2
  Constant : Constant  Value=trim_control
  Demux : Demux
  Demux1 : Demux  Outputs=3
  Demux2 : Demux  Outputs=3
  Demux3 : Demux  Outputs=3
  Display : Display
  Gain : Gain  Gain=1000
  IBVS Conroller : MATLAB Function  TreatAsAtomicUnit=on
  Image Error Scope : Display
  Integrator : Integrator
  Integrator1 : Integrator
  Integrator2 : Integrator
  Ki : Gain  Gain=Ki  Multiplication=Matrix(K*u) (u vector)
  Kp : Gain  Gain=Kp  Multiplication=Matrix(K*u) (u vector)
  Mux : Mux
  Mux1 : Mux  Inputs=3
  Mux3 : Mux  Inputs=3
  Saturation : Saturate  UpperLimit=15  LowerLimit=-15
  Sum : Sum  Inputs=|++
  Sum3 : Sum  Inputs=+|-
  To Workspace : ToWorkspace  VariableName=E_imag  SampleTime=-1
  ex&ey : Scope  NumInputPorts=2
  u_v : Display
  z : Scope
  U : Outport
  wires:
  Mux3/1 -> Ki/1
  F16State/1 -> IBVS Conroller/4(F16State), Kp/1, Display/1
  Integrator/1 -> Mux3/1
  Demux1/3 -> Integrator2/1  "Vx"
  Integrator2/1 -> Mux3/3
  Demux1/1 -> Saturation/1  "Vz"
  Ki/1 -> Sum3/1
  Kp/1 -> Sum3/2
  Sum3/1 -> Demux/1
  Saturation/1 -> Integrator/1
  Demux/2 -> Mux/2  "q"
  Demux/3 -> Mux/3  "p"
  Demux/4 -> Mux/4  "r"
  Demux/1 -> Gain/1
  Gain/1 -> Mux/1  "ft"
  Constant/1 -> Sum/2
  Mux/1 -> Sum/1
  Sum/1 -> U/1
  Demux2/1 -> IBVS Conroller/1(Z)
  Demux2/2 -> IBVS Conroller/2(ex)
  Demux2/3 -> IBVS Conroller/3(ey)
  IBVS Conroller/2(u_vcy) -> Mux1/2
  IBVS Conroller/1(u_vcz) -> Mux1/1
  IBVS Conroller/3(u_vcx) -> Mux1/3
  Mux1/1 -> u_v/1, Demux1/1
  Image Error/1 -> To Workspace/1, Demux3/1, Image Error Scope/1, Demux2/1
  Demux3/2 -> ex&ey/1
  Demux1/2 -> Integrator1/1  "Vy"
  Integrator1/1 -> Mux3/2
  Demux3/1 -> z/1
  Demux3/3 -> ex&ey/2

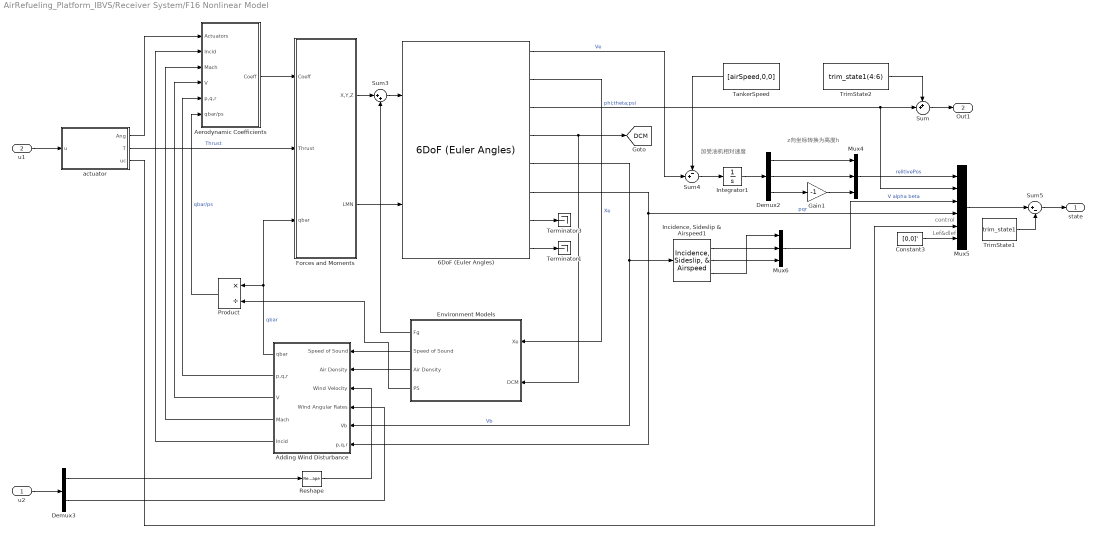
== system AirRefueling_Platform_IBVS/Receiver System/F16 Nonlinear Model ==
  note: 加受油机相对速度
  note: z向坐标转换为高度h
  note: Lef&dlef
  note: control
  u2 : Inport
  u1 : Inport  Port=2
  6DoF (Euler Angles) : aerolibobsolete/6DoF (Euler Angles)  units=English (Velocity in ft/s)  mtype=Fixed  rep=Euler Angles  xme_0=xyz_0  Vm_0=uvw_0  eul_0=Euler_0  pm_0=pqr_0  mass_0=mass  mass_e=0.5  mass_f=2.0  inertia=Inertia  inertia_e=eye(3)  inertia_f=2*eye(3)  k_quat=1.0
  Adding Wind Disturbance : Subsystem
  Aerodynamic Coefficients : Subsystem
  Constant3 : Constant  Value=[0,0]'
  Demux2 : Demux  Outputs=3
  Demux3 : Demux  Outputs=2
  Environment Models : Subsystem
  Forces and Moments : Subsystem
  Gain1 : Gain  Gain=-1
  "Incidence, Sideslip & Airspeed1" : aerolibasang/Incidence, Sideslip, & Airspeed
  Integrator1 : Integrator
  Mux4 : Mux  Inputs=3
  Mux5 : Mux  Inputs=6
  Mux6 : Mux  Inputs=3
  Product : Product  Inputs=*/  InputSameDT=on  SaturateOnIntegerOverflow=on  OutDataTypeStr=Inherit: Same as first input
  Reshape : Reshape
  Sum : Sum  Inputs=++|
  Sum3 : Sum  Inputs=|++  InputSameDT=on  SaturateOnIntegerOverflow=on  OutDataTypeStr=Inherit: Same as first input
  Sum4 : Sum  Inputs=-+|
  Sum5 : Sum  Inputs=|+-
  TankerSpeed : Constant  Value=[airSpeed,0,0]
  Terminator1 : Terminator
  Terminator3 : Terminator
  TrimState1 : Constant  Value=trim_state1
  TrimState2 : Constant  Value=trim_state1(4:6)
  actuator : Subsystem
  state : Outport
  Out1 : Outport  Port=2
  tag scope: DCM=global
  wires:
  6DoF (Euler Angles)/8 -> Terminator1/1
  6DoF (Euler Angles)/7 -> Terminator3/1
  6DoF (Euler Angles)/4 -> Environment Models/2(DCM), [DCM]
  Adding Wind Disturbance/5(Incid) -> Aerodynamic Coefficients/2(Incid)
  Aerodynamic Coefficients/1(Coeff) -> Forces and Moments/1(Coeff)
  Environment Models/2(Speed of Sound) -> Adding Wind Disturbance/1(Speed of Sound)
  Environment Models/3(Air Density) -> Adding Wind Disturbance/2(Air Density)
  Forces and Moments/2(LMN) -> 6DoF (Euler Angles)/2
  Adding Wind Disturbance/1(qbar) -> Forces and Moments/3(qbar), Product/1  "qbar"
  Forces and Moments/1(X,Y,Z) -> Sum3/1
  Sum3/1 -> 6DoF (Euler Angles)/1
  Environment Models/1(Fg) -> Sum3/2
  Adding Wind Disturbance/3(V) -> Aerodynamic Coefficients/4(V)
  Adding Wind Disturbance/4(Mach) -> Aerodynamic Coefficients/3(Mach)
  Adding Wind Disturbance/2("p,q,r ") -> Aerodynamic Coefficients/5(p,q,r)
  Environment Models/4(PS) -> Product/2
  Product/1 -> Aerodynamic Coefficients/6(qbar/ps)  "qbar/ps"
  u1/1 -> actuator/1(u)
  actuator/2(T) -> Forces and Moments/2(Thrust)  "Thrust"
  actuator/1(Ang) -> Aerodynamic Coefficients/1(Actuators)
  6DoF (Euler Angles)/3 -> Mux5/2, Sum/2  "phi;theta;psi"
  "Incidence, Sideslip & Airspeed1"/1 -> Mux6/2
  "Incidence, Sideslip & Airspeed1"/2 -> Mux6/3
  Mux6/1 -> Mux5/3  "V alpha beta"
  "Incidence, Sideslip & Airspeed1"/3 -> Mux6/1
  6DoF (Euler Angles)/6 -> Adding Wind Disturbance/6(p,q,r), Mux5/4  "pqr"
  6DoF (Euler Angles)/5 -> Adding Wind Disturbance/5(Vb), "Incidence, Sideslip & Airspeed1"/1  "Vb"
  Mux5/1 -> Sum5/1
  TrimState1/1 -> Sum5/2
  Sum5/1 -> state/1
  actuator/3(uc) -> Mux5/5
  Constant3/1 -> Mux5/6
  Demux2/2 -> Mux4/2
  Demux2/3 -> Gain1/1
  Mux4/1 -> Mux5/1  "relitivePos"
  Demux2/1 -> Mux4/1
  Gain1/1 -> Mux4/3
  Sum4/1 -> Integrator1/1
  Integrator1/1 -> Demux2/1
  6DoF (Euler Angles)/2 -> Environment Models/1(Xe)  "Xe"
  u2/1 -> Demux3/1
  Reshape/1 -> Adding Wind Disturbance/3(Wind Velocity)
  Demux3/1 -> Reshape/1
  Sum/1 -> Out1/1
  Demux3/2 -> Adding Wind Disturbance/4(Wind Angular Rates)
  TrimState2/1 -> Sum/1
  6DoF (Euler Angles)/1 -> Sum4/2  "Ve"
  TankerSpeed/1 -> Sum4/1

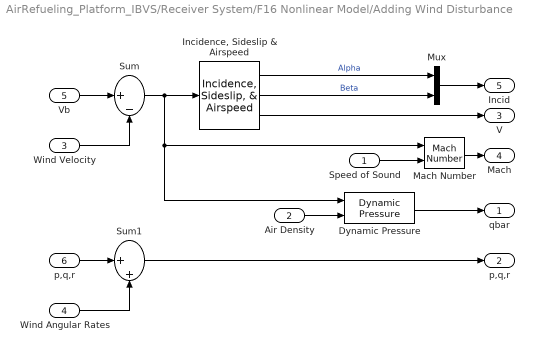
== system AirRefueling_Platform_IBVS/Receiver System/F16 Nonlinear Model/Adding Wind Disturbance ==
  Speed of Sound : Inport
  Air Density : Inport  Port=2
  Wind Velocity : Inport  Port=3  PortDimensions=3
  Wind Angular Rates : Inport  Port=4  PortDimensions=3
  Vb : Inport  Port=5  PortDimensions=3
  p,q,r : Inport  Port=6  PortDimensions=3
  Dynamic Pressure : aerolibasang/Dynamic Pressure
  "Incidence, Sideslip & Airspeed" : aerolibasang/Incidence, Sideslip, & Airspeed
  Mach Number : aerolibasang/Mach Number
  Mux : Mux  Inputs=2
  Sum : Sum  Inputs=|+-  InputSameDT=on  SaturateOnIntegerOverflow=on  OutDataTypeStr=Inherit: Same as first input
  Sum1 : Sum  Inputs=|++  InputSameDT=on  SaturateOnIntegerOverflow=on  OutDataTypeStr=Inherit: Same as first input
  qbar : Outport  InitialOutput=0
  "p,q,r " : Outport  Port=2
  V : Outport  Port=3
  Mach : Outport  Port=4
  Incid : Outport  Port=5
  wires:
  "Incidence, Sideslip & Airspeed"/3 -> V/1
  Dynamic Pressure/1 -> qbar/1
  Air Density/1 -> Dynamic Pressure/2
  Mach Number/1 -> Mach/1
  Sum/1 -> Dynamic Pressure/1, Mach Number/1, "Incidence, Sideslip & Airspeed"/1
  Vb/1 -> Sum/1
  Speed of Sound/1 -> Mach Number/2
  Wind Velocity/1 -> Sum/2
  "Incidence, Sideslip & Airspeed"/2 -> Mux/2  "Beta"
  Mux/1 -> Incid/1
  "Incidence, Sideslip & Airspeed"/1 -> Mux/1  "Alpha"
  p,q,r/1 -> Sum1/1
  Wind Angular Rates/1 -> Sum1/2
  Sum1/1 -> "p,q,r "/1

== system AirRefueling_Platform_IBVS/Receiver System/F16 Nonlinear Model/Aerodynamic Coefficients ==
  Actuators : Inport
  Incid : Inport  Port=2
  Mach : Inport  Port=3
  V : Inport  Port=4
  p,q,r : Inport  Port=5
  qbar/ps : Inport  Port=6
  Angle Conversion : aerolibconvert2/Angle Conversion  IU=rad  OU=deg
  Interpreted MATLAB Function : MATLABFcn  MATLABFcn=F16Coef1  OutputDimensions=6
  Leading Edge Flap : Subsystem
  Mux : Mux  Inputs=6
  Terminator2 : Terminator
  alpha : Selector  InputPortWidth=2  IndexOptions=Index vector (dialog)  Indices=1  OutputSizes=1
  flag : Constant  Value=fi_flag
  Coeff : Outport  InitialOutput=0
  wires:
  Angle Conversion/1 -> alpha/1, Mux/2
  Incid/1 -> Angle Conversion/1
  qbar/ps/1 -> Leading Edge Flap/2(qbar/ps)
  alpha/1 -> Leading Edge Flap/1(alpha)
  V/1 -> Mux/1
  p,q,r/1 -> Mux/3
  Actuators/1 -> Mux/4
  flag/1 -> Mux/5
  Mach/1 -> Terminator2/1
  Interpreted MATLAB Function/1 -> Coeff/1
  Mux/1 -> Interpreted MATLAB Function/1
  Leading Edge Flap/1(delta_lef (deg)) -> Mux/6

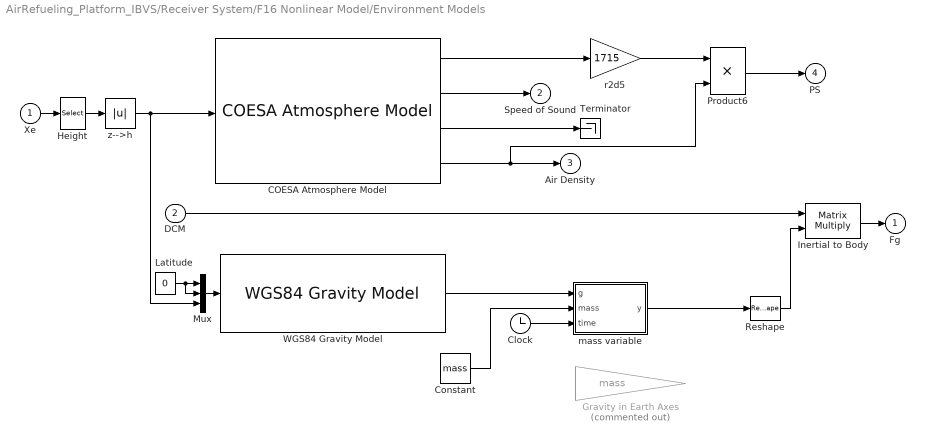
== system AirRefueling_Platform_IBVS/Receiver System/F16 Nonlinear Model/Environment Models ==
  Xe : Inport  PortDimensions=3
  DCM : Inport  Port=2
  COESA Atmosphere Model : aerolibatmos2/COESA Atmosphere Model  units=English (Velocity in ft/s)  spec=1976 COESA-extended U.S. Standard Atmosphere  model=Profile  profile_var=High temperature  profile_percent=10%  profile_alt=5 km (16404 ft)  envelope_var=High temperature  envelope_percent=1%  action=None
  Clock : Clock
  Constant : Constant  Value=mass
  Gravity in Earth Axes : Gain  Commented=on  Gain=mass  SaturateOnIntegerOverflow=on  OutDataTypeStr=Inherit: Same as input  ParamDataTypeStr=Inherit: Same as input
  Height : Selector  InputPortWidth=3  IndexOptions=Index vector (dialog)  Indices=[3]  OutputSizes=1
  Inertial to Body : Product  Multiplication=Matrix(*)  InputSameDT=on  SaturateOnIntegerOverflow=on  OutDataTypeStr=Inherit: Same as first input
  Latitude : Constant  Value=0
  Mux : Mux  Inputs=3
  Product6 : Product  Inputs=**  InputSameDT=on  SaturateOnIntegerOverflow=on  OutDataTypeStr=Inherit: Same as first input
  Reshape : Reshape
  Terminator : Terminator
  "WGS84 Gravity Model " : aerolibobsolete/WGS84 Gravity Model   model=WGS84 Taylor Series  units=English  no_atmos=on  precessing=on  jd_loc=off  month=October  day=10  year=2004  no_centrifugal=on  action=None
  mass variable : MATLAB Function  TreatAsAtomicUnit=on
  r2d5 : Gain  Gain=1715  SaturateOnIntegerOverflow=on  OutDataTypeStr=Inherit: Same as input  ParamDataTypeStr=Inherit: Same as input
  z-->h : Abs
  Fg : Outport  InitialOutput=0
  Speed of Sound : Outport  Port=2  InitialOutput=0
  Air Density : Outport  Port=3  InitialOutput=0
  PS : Outport  Port=4
  wires:
  Reshape/1 -> Inertial to Body/2
  Mux/1 -> "WGS84 Gravity Model "/1
  z-->h/1 -> Mux/3, COESA Atmosphere Model/1
  COESA Atmosphere Model/2 -> Speed of Sound/1
  COESA Atmosphere Model/3 -> Terminator/1
  Height/1 -> z-->h/1
  Xe/1 -> Height/1
  Latitude/1 -> Mux/2, Mux/1
  "WGS84 Gravity Model "/1 -> mass variable/1(g)
  mass variable/1(y) -> Reshape/1
  DCM/1 -> Inertial to Body/1
  Inertial to Body/1 -> Fg/1
  COESA Atmosphere Model/4 -> Product6/2, Air Density/1
  COESA Atmosphere Model/1 -> r2d5/1
  Product6/1 -> PS/1
  r2d5/1 -> Product6/1
  Clock/1 -> mass variable/3(time)
  Constant/1 -> mass variable/2(mass)

== system AirRefueling_Platform_IBVS/Receiver System/F16 Nonlinear Model/Forces and Moments ==
  Coeff : Inport
  Thrust : Inport  Port=2
  qbar : Inport  Port=3
  "Aerodynamic Forces and Moments " : aerolibadyn/Aerodynamic Forces and Moments   inputAxes=Body  outputForceAxes=Body  outputMomentAxes=Body  S=S_ref  b=b_ref  cbar=d_ref
  Center of Gravity : Constant  Value=[-0 0 0]
  Center of Pressure : Constant  Value=[-0 0 0]
  Sum : Sum  Inputs=++|  InputSameDT=on  SaturateOnIntegerOverflow=on  OutDataTypeStr=Inherit: Same as first input
  X,Y,Z : Outport  InitialOutput=0
  LMN : Outport  Port=2  InitialOutput=0
  wires:
  Center of Pressure/1 -> "Aerodynamic Forces and Moments "/4
  Center of Gravity/1 -> "Aerodynamic Forces and Moments "/3
  "Aerodynamic Forces and Moments "/1 -> Sum/2
  "Aerodynamic Forces and Moments "/2 -> LMN/1
  Sum/1 -> X,Y,Z/1
  Thrust/1 -> Sum/1
  qbar/1 -> "Aerodynamic Forces and Moments "/2
  Coeff/1 -> "Aerodynamic Forces and Moments "/1

== system AirRefueling_Platform_IBVS/Receiver System/F16 Nonlinear Model/actuator ==
  u : Inport
  Aileron Actuator : Subsystem
  Demux : Demux
  Elevator Actuator : Subsystem
  Mux : Mux  Inputs=2
  Mux1 : Mux  Inputs=3
  Mux2 : Mux  Inputs=3
  Rudder Actuator : Subsystem
  Thrust Model : Subsystem
  Ty : Constant  Value=0
  Tz : Constant  Value=0
  Ang : Outport
  T : Outport  Port=2
  uc : Outport  Port=3
  wires:
  u/1 -> Demux/1
  Mux2/1 -> Ang/1, Mux/2
  Thrust Model/1(T) -> Mux/1, Mux1/1  "Tx"
  Ty/1 -> Mux1/2
  Tz/1 -> Mux1/3
  Mux1/1 -> T/1
  Mux/1 -> uc/1
  Demux/1 -> Thrust Model/1(delta_t)
  Elevator Actuator/1(el) -> Mux2/1  "el"
  Aileron Actuator/1(ail) -> Mux2/2  "ail"
  Rudder Actuator/1(rud) -> Mux2/3  "rud"
  Demux/2 -> Elevator Actuator/1(delta_e)
  Demux/3 -> Aileron Actuator/1(delta_a)
  Demux/4 -> Rudder Actuator/1(delta_r)

== system AirRefueling_Platform_IBVS/Receiver System/F16 Nonlinear Model/Aerodynamic Coefficients/Leading Edge Flap ==
  note: see NASA Technical Paper 1538, p34
  note: Initialize LF_state with -alpha0 value in degrees!!!!
  alpha : Inport
  qbar/ps : Inport  Port=2
  Gain : Gain  Gain=2  SaturateOnIntegerOverflow=on  OutDataTypeStr=Inherit: Same as input  ParamDataTypeStr=Inherit: Same as input
  Gain1 : Gain  Gain=7.25  SaturateOnIntegerOverflow=on  OutDataTypeStr=Inherit: Same as input  ParamDataTypeStr=Inherit: Same as input
  Gain2 : Gain  Gain=1.38  SaturateOnIntegerOverflow=on  OutDataTypeStr=Inherit: Same as input  ParamDataTypeStr=Inherit: Same as input
  LEF Actuator : Subsystem
  LF_state : Integrator  InitialCondition=-alpha0
  Sum : Sum  Inputs=-|+|+  InputSameDT=on  SaturateOnIntegerOverflow=on  OutDataTypeStr=Inherit: Same as first input
  Sum1 : Sum  Inputs=|+-  InputSameDT=on  SaturateOnIntegerOverflow=on  OutDataTypeStr=Inherit: Same as first input
  Sum2 : Sum  Inputs=++|  InputSameDT=on  SaturateOnIntegerOverflow=on  OutDataTypeStr=Inherit: Same as first input
  coeff1 : Constant  Value=1.45
  lef Saturation : Saturate  UpperLimit=25  LowerLimit=0
  r2d6 : Gain  Gain=9.05  SaturateOnIntegerOverflow=on  OutDataTypeStr=Inherit: Same as input  ParamDataTypeStr=Inherit: Same as input
  delta_lef (deg) : Outport
  wires:
  Sum1/1 -> Gain1/1
  Gain1/1 -> LF_state/1
  Gain/1 -> Sum2/1
  Gain2/1 -> Sum/2
  coeff1/1 -> Sum/3
  Sum2/1 -> Sum1/2, Gain2/1
  LF_state/1 -> Sum2/2
  alpha/1 -> Sum1/1, Gain/1
  qbar/ps/1 -> r2d6/1
  r2d6/1 -> Sum/1
  lef Saturation/1 -> delta_lef (deg)/1
  Sum/1 -> LEF Actuator/1(dlef)
  LEF Actuator/1(LEF) -> lef Saturation/1

== system AirRefueling_Platform_IBVS/Receiver System/F16 Nonlinear Model/actuator/Aileron Actuator ==
  delta_a : Inport
  Command Saturation : Saturate  UpperLimit=21.5  LowerLimit=-21.5
  Gain : Gain  Gain=20.2  SaturateOnIntegerOverflow=on  OutDataTypeStr=Inherit: Same as input  ParamDataTypeStr=Inherit: Same as input
  "Integrator " : Integrator  InitialCondition=trim_ail  UpperSaturationLimit=21.5  LowerSaturationLimit=-21.5
  Rate Saturation : Saturate  UpperLimit=80  LowerLimit=-80
  Sum : Sum  Inputs=|+-  InputSameDT=on  SaturateOnIntegerOverflow=on  OutDataTypeStr=Inherit: Same as first input
  ail : Outport
  wires:
  delta_a/1 -> Command Saturation/1
  "Integrator "/1 -> ail/1, Sum/2
  Sum/1 -> Gain/1
  Gain/1 -> Rate Saturation/1
  Command Saturation/1 -> Sum/1
  Rate Saturation/1 -> "Integrator "/1

== system AirRefueling_Platform_IBVS/Receiver System/F16 Nonlinear Model/actuator/Elevator Actuator ==
  delta_e : Inport
  Command Saturation : Saturate  UpperLimit=25  LowerLimit=-25
  Gain : Gain  Gain=20.2  SaturateOnIntegerOverflow=on  OutDataTypeStr=Inherit: Same as input  ParamDataTypeStr=Inherit: Same as input
  "Integrator " : Integrator  InitialCondition=trim_ele  UpperSaturationLimit=25  LowerSaturationLimit=-25
  Rate Saturation : Saturate  UpperLimit=60  LowerLimit=-60
  Sum : Sum  Inputs=|+-  InputSameDT=on  SaturateOnIntegerOverflow=on  OutDataTypeStr=Inherit: Same as first input
  el : Outport
  wires:
  delta_e/1 -> Command Saturation/1
  Command Saturation/1 -> Sum/1
  Sum/1 -> Gain/1
  Gain/1 -> Rate Saturation/1
  "Integrator "/1 -> el/1, Sum/2
  Rate Saturation/1 -> "Integrator "/1

== system AirRefueling_Platform_IBVS/Receiver System/F16 Nonlinear Model/actuator/Rudder Actuator ==
  delta_r : Inport
  Command Saturation : Saturate  UpperLimit=30  LowerLimit=-30
  Gain : Gain  Gain=20.2  SaturateOnIntegerOverflow=on  OutDataTypeStr=Inherit: Same as input  ParamDataTypeStr=Inherit: Same as input
  "Integrator " : Integrator  InitialCondition=trim_rud  UpperSaturationLimit=30  LowerSaturationLimit=-30
  Rate Saturation : Saturate  UpperLimit=120  LowerLimit=-120
  Sum : Sum  Inputs=|+-  InputSameDT=on  SaturateOnIntegerOverflow=on  OutDataTypeStr=Inherit: Same as first input
  rud : Outport
  wires:
  "Integrator "/1 -> rud/1, Sum/2
  Sum/1 -> Gain/1
  delta_r/1 -> Command Saturation/1
  Rate Saturation/1 -> "Integrator "/1
  Gain/1 -> Rate Saturation/1
  Command Saturation/1 -> Sum/1

== system AirRefueling_Platform_IBVS/Receiver System/F16 Nonlinear Model/actuator/Thrust Model ==
  delta_t : Inport
  Command Saturation : Saturate  UpperLimit=19000  LowerLimit=1000
  Gain : Gain  SaturateOnIntegerOverflow=on  OutDataTypeStr=Inherit: Same as input  ParamDataTypeStr=Inherit: Same as input
  "Integrator " : Integrator  InitialCondition=trim_thrust  UpperSaturationLimit=30  LowerSaturationLimit=-30
  Rate Saturation : Saturate  UpperLimit=10000  LowerLimit=-10000
  Sum : Sum  Inputs=|+-  InputSameDT=on  SaturateOnIntegerOverflow=on  OutDataTypeStr=Inherit: Same as first input
  T : Outport
  wires:
  delta_t/1 -> Command Saturation/1
  Gain/1 -> Rate Saturation/1
  "Integrator "/1 -> T/1, Sum/2
  Command Saturation/1 -> Sum/1
  Sum/1 -> Gain/1
  Rate Saturation/1 -> "Integrator "/1

== system AirRefueling_Platform_IBVS/Receiver System/F16 Nonlinear Model/Aerodynamic Coefficients/Leading Edge Flap/LEF Actuator ==
  dlef : Inport
  Command Saturation : Saturate  UpperLimit=25  LowerLimit=0
  Gain3 : Gain  Gain=1/0.136  SaturateOnIntegerOverflow=on  OutDataTypeStr=Inherit: Same as input  ParamDataTypeStr=Inherit: Same as input
  "Integrator " : Integrator  InitialCondition=dLEF  UpperSaturationLimit=21.5  LowerSaturationLimit=-21.5
  Rate Saturation : Saturate  UpperLimit=25  LowerLimit=-25
  Sum3 : Sum  Inputs=|+-  InputSameDT=on  SaturateOnIntegerOverflow=on  OutDataTypeStr=Inherit: Same as first input
  LEF : Outport
  wires:
  Gain3/1 -> Rate Saturation/1
  Rate Saturation/1 -> "Integrator "/1
  "Integrator "/1 -> LEF/1, Sum3/2
  Sum3/1 -> Gain3/1
  dlef/1 -> Command Saturation/1
  Command Saturation/1 -> Sum3/1

== matlab function AirRefueling_Platform_IBVS/Original IBVS/Controller/controller  ==
  data: y output
function y = fcn()

y = 0;

== matlab function AirRefueling_Platform_IBVS/Visual Servo Block/MATLAB Function ==
  data: u input; y output
function y = fcn(u)
%#codegen

 Ir=u(:,:,1)*2-u(:,:,2)*1-u(:,:,3)*1;

% Ir=u(:,:,1)*0.3-u(:,:,2)*0.59-u(:,:,3)*0.11

S=size(Ir);
Iin=zeros(S(1),S(2));
for i=1:S(1)
    for j=1:S(2)
       if Ir(i,j)<50
            Iin(i,j)=0;
        else
            Iin(i,j)=1;
        end
    end
end


y = Iin;

== matlab function AirRefueling_Platform_IBVS/Tanker System/   ==
  data: u input; y output
function y = WindTurFromTank(u)
%#codegen

y = TankerVortexWindField(u);
